simulink model "working_model_of_actual_car"  (Simulink 7.7)
settings: Solver=ode45  StartTime=0.0  StopTime=1200  RelTol=1e-3
values from neighbouring files (symbols this model uses):
  b1 = 500    [initialise_parameters.m]
  b2 = 1500    [initialise_parameters.m]
  k1 = 60000*4    (= 240000)    [initialise_parameters.m]
  k2 = 1350000*4    (= 5400000)    [initialise_parameters.m]
  m1 = 500    [initialise_parameters.m]
  m2 = 50    [initialise_parameters.m]
settings Model: Creator=Rohan  LastModifiedBy=Rohan
settings DataIOCC: ExternalInput=[Zposn(1),Zposn(2)]  LoadExternalInput=on

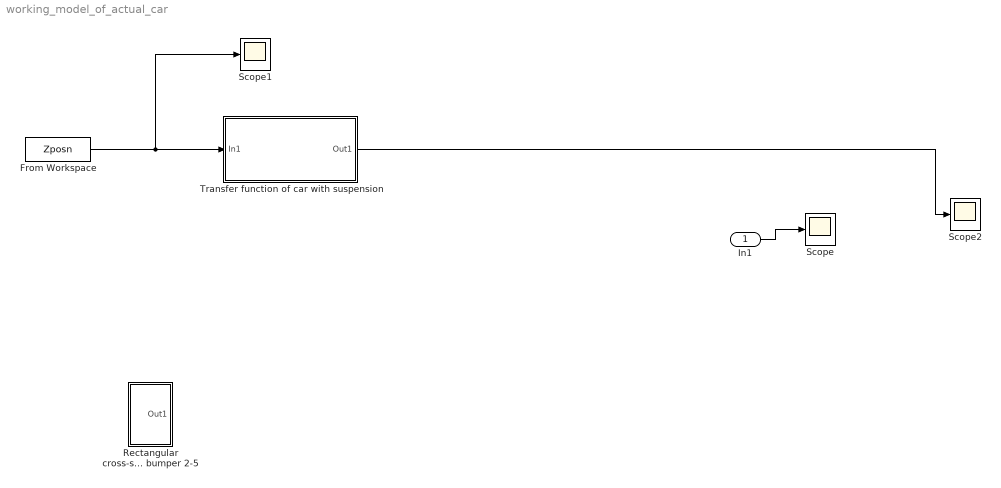
== system working_model_of_actual_car ==
  In1 : Inport
  From Workspace : FromWorkspace  VariableName=Zposn  SampleTime=0
  Rectangular cross-section bumper 2-5 : Subsystem
  Scope : Scope
  Scope1 : Scope
  Scope2 : Scope
      settings: YMin=-90  YMax=25  SaveName=ScopeData2
  Transfer function of car with suspension : Subsystem
  wires:
  In1/1 -> Scope/1
  Transfer function of car with suspension/1(Out1) -> Scope2/1
  From Workspace/1 -> Transfer function of car with suspension/1(In1), Scope1/1

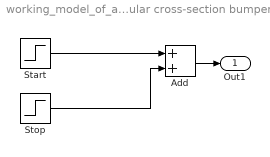
== system working_model_of_actual_car/Rectangular cross-section bumper 2-5 ==
  Add : Sum
  Start : Step  Time=2  SampleTime=0
  Stop : Step  Time=5  After=-1  SampleTime=0
  Out1 : Outport
  wires:
  Stop/1 -> Add/2
  Start/1 -> Add/1
  Add/1 -> Out1/1

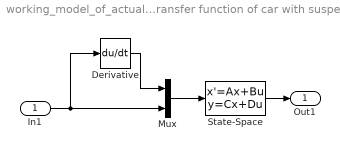
== system working_model_of_actual_car/Transfer function of car with suspension ==
  In1 : Inport
  Derivative : Derivative
  Mux : Mux  Inputs=2
  State-Space : StateSpace  A=[-b1/m1 b1/m1 -k1/m1 k1/m1; b1/m1 -(b1+b2)/m2 k1/m1 -(k1+k2)/m2;1 0 0 0; 0 1 0 0]  B=[0 0; b2/m2 k2/m2;0 0;0 0]  C=[0 0 1 0; 0 0 0 1; 0 0 1 -1]  D=[0 0;0 0;0 0]
  Out1 : Outport
  wires:
  Mux/1 -> State-Space/1
  Derivative/1 -> Mux/1
  In1/1 -> Derivative/1, Mux/2
  State-Space/1 -> Out1/1
